simulink model "Exemplo_Suspensao"  (R2015a)
settings: Solver=ode3  StartTime=0.0  StopTime=inf  FixedStep=0.1  MaxStep=1  RelTol=1e-3
libraries: simulink x2, AvgModels x1
settings Model: CovSFcnEnable=off  Creator=lgalotto  LastModifiedBy=lgalo
settings DataIOCC: SignalLoggingSaveFormat=ModelDataLogs
settings OptimizationCC: ExpressionDepthLimit=2147483647
settings DebuggingCC: UnderspecifiedInitializationDetection=Classic  MergeDetectMultiDrivingBlocksExec=none  SolverPrmCheckMsg=warning  FcnCallInpInsideContextMsg=EnableAllAsWarning  StateNameClashWarn=warning
settings GRTTargetCC: CombineOutputUpdateFcns=off  GRTInterface=on

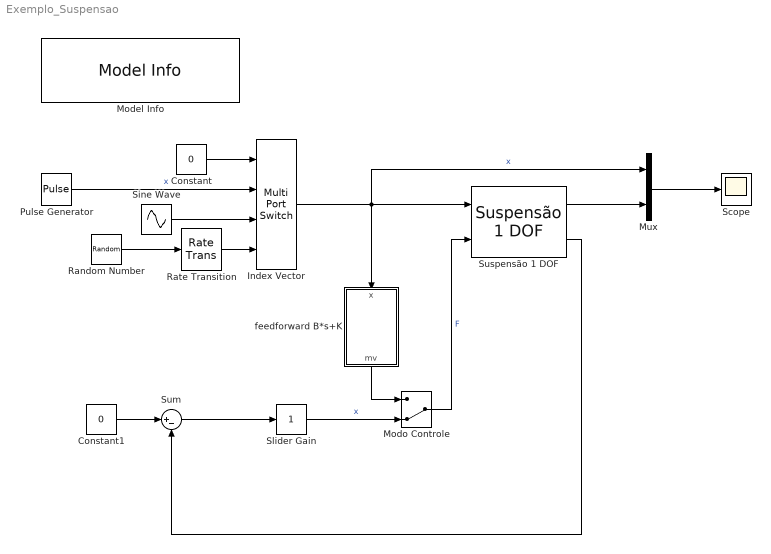
== system Exemplo_Suspensao ==
  Constant : Constant  Value=0
  Constant1 : Constant  Value=0
  Index Vector : MultiPortSwitch  DataPortOrder=Zero-based contiguous  zeroidx=on
  Model Info : simulink/Model-Wide Utilities/Model Info  Frame=on  DisplayStringWithTags=|  HorizontalTextAlignment=Center  LeftAlignmentValue=0.5  SourceBlockDiagram=Exemplo_Suspensao  TagMaxNumber=20
      | Exemplo de Controle de Suspensão
      | Prof Luigi Galotto Jr
      | %<ModifiedDate>
      | %<Description>
  Modo Controle : ManualSwitch  CurrentSetting=0
  Mux : Mux  Inputs=2
  Pulse Generator : DiscretePulseGenerator  PulseType=Time based  Period=100  PulseWidth=50
  Random Number : RandomNumber  Variance=0.5  SampleTime=5
  Rate Transition : RateTransition
  Scope : Scope
  Sine Wave : Sin  SampleTime=0
  Slider Gain : simulink/Math Operations/Slider Gain  low=0  gain=1  high=2
  Sum : Sum  Inputs=|+-
  Suspensão 1 DOF : AvgModels/Modelos Animados/Suspensão 1 DOF  M=500  K=10  B=50
  feedforward B*s+K : Subsystem
  wires:
  Index Vector/1 -> feedforward B*s+K/1(x), Suspensão 1 DOF/1, Mux/1  "x"
  Pulse Generator/1 -> Index Vector/2  "x"
  Constant/1 -> Index Vector/1
  Sine Wave/1 -> Index Vector/3
  Random Number/1 -> Rate Transition/1
  Sum/1 -> Slider Gain/1
  Constant1/1 -> Sum/1
  Rate Transition/1 -> Index Vector/4
  Suspensão 1 DOF/1 -> Mux/2
  feedforward B*s+K/1(mv) -> Modo Controle/1
  Suspensão 1 DOF/2 -> Sum/2
  Mux/1 -> Scope/1
  Slider Gain/1 -> Modo Controle/2  "x"
  Modo Controle/1 -> Suspensão 1 DOF/2  "F"

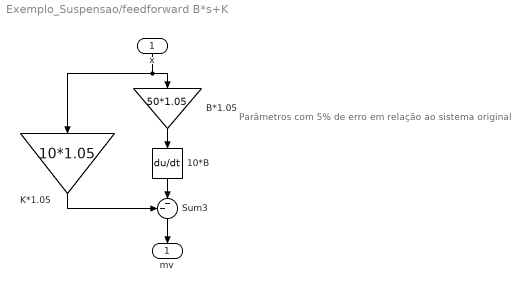
== system Exemplo_Suspensao/feedforward B*s+K ==
  note: Parâmetros com 5% de erro em relação ao sistema original
  x : Inport
  10*B : Derivative  CoefficientInTFapproximation=10*50
  B*1.05 : Gain  Gain=50*1.05
  K*1.05 : Gain  Gain=10*1.05
  Sum3 : Sum  Inputs=--|
  mv : Outport
  wires:
  10*B/1 -> Sum3/2
  K*1.05/1 -> Sum3/1
  B*1.05/1 -> 10*B/1
  x/1 -> B*1.05/1, K*1.05/1
  Sum3/1 -> mv/1
